simulink model "DataDriven_Sim"  (R2019a)
settings: Solver=ode4  StartTime=0.0  StopTime=40  FixedStep=0.005  MaxStep=0.2  RelTol=1e-3
values from neighbouring files (symbols this model uses):
  n = size(A,1)    [getMPC.m]    (also in poolData.m = size(yin,1); poolDataLIST.m = size(yin,1); poolData_EDMD.m = size(yin,1); solveMPCprob.m)
  nObsv = size(A,1)    [linearizeData.m]
  polyorder = p.polyorder    [sparseGalerkinControl_Discrete.m]
  polysine = p.polysine    [sparseGalerkinControl_Discrete.m]
  usesine = p.usesine    [sparseGalerkinControl_Discrete.m]
undefined symbols (not defined in the file or in its folder): F, Fi, lqi_, lqr_, param, ref_stab, ref_track, sigbuilder_block, stab, track
libraries: simulink x1
settings Model: Creator=yashasvi_sai  LastModifiedBy=ICS
settings SolverCC: ZeroCrossAlgorithm=Adaptive
settings DebuggingCC: IgnoredZcDiagnostic=none

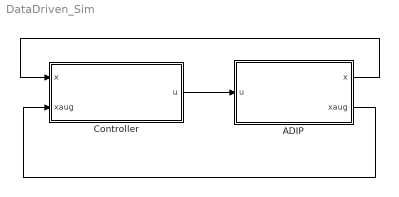
== system DataDriven_Sim ==
  ADIP : Subsystem
  Controller : Subsystem
  wires:
  ADIP/2(xaug) -> Controller/2(xaug)
  ADIP/1(x) -> Controller/1(x)
  Controller/1(u) -> ADIP/1(u)

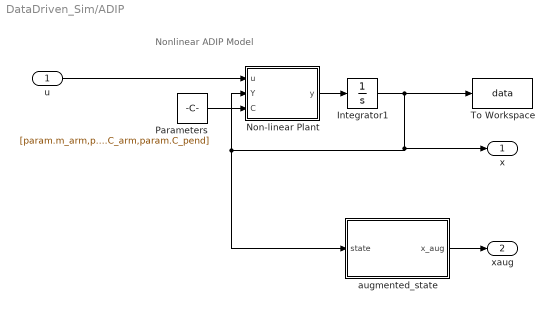
== system DataDriven_Sim/ADIP ==
  note: Nonlinear ADIP Model
  u : Inport
  Integrator1 : Integrator  InitialCondition=param.theta0
  "Non-linear Plant " : MATLAB Function  TreatAsAtomicUnit=on
  Parameters : Constant  Value=[param.m_arm,param.m_pend,param.m_hinge,param.l_pivot,param.l_pend,param.g,param.Jarm,param.Jpend,param.Jl,param.Jhinge, param.C_arm,param.C_pend]
  To Workspace : ToWorkspace  VariableName=data  SampleTime=-1
  augmented_state : Subsystem
  x : Outport
  xaug : Outport  Port=2
  wires:
  "Non-linear Plant "/1(y) -> Integrator1/1
  Integrator1/1 -> augmented_state/1(state), "Non-linear Plant "/2(Y), x/1, To Workspace/1
  u/1 -> "Non-linear Plant "/1(u)
  Parameters/1 -> "Non-linear Plant "/3(C)
  augmented_state/1(x_aug) -> xaug/1

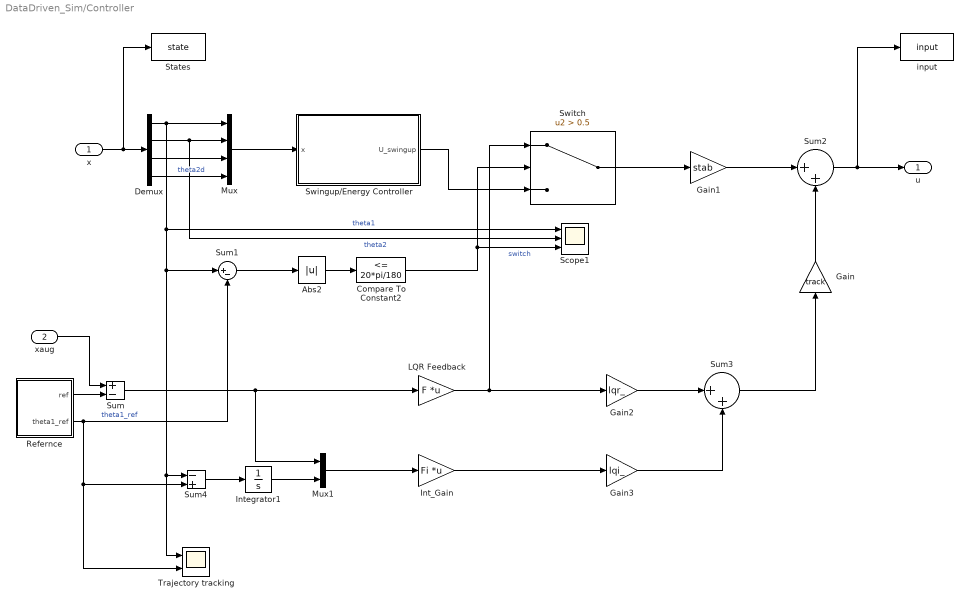
== system DataDriven_Sim/Controller ==
  x : Inport
  xaug : Inport  Port=2
  Abs2 : Abs
  Compare To Constant2 : simulink/Logic and Bit Operations/Compare To Constant  relop=<=  const=20*pi/180  OutDataTypeStr=boolean
  Demux : Demux
  Gain : Gain  Gain=track
  Gain1 : Gain  Gain=stab
  Gain2 : Gain  Gain=lqr_
  Gain3 : Gain  Gain=lqi_
  Int_Gain : Gain  Gain=Fi  Multiplication=Matrix(K*u)
  Integrator1 : Integrator
  LQR Feedback : Gain  Gain=F  Multiplication=Matrix(K*u)
  Mux : Mux
  Mux1 : Mux  Inputs=2
  Refernce : Subsystem
  Scope1 : Scope  NumInputPorts=3
  States : ToWorkspace  VariableName=state  SampleTime=-1
  Sum : Sum  Inputs=+-
  Sum1 : Sum  Inputs=|+-
  Sum2 : Sum  Inputs=|++
  Sum3 : Sum  Inputs=|++
  Sum4 : Sum  Inputs=-+
  Swingup/Energy Controller : Subsystem
  Switch : Switch  Criteria=u2 > Threshold  Threshold=0.5
  Trajectory tracking : Scope  NumInputPorts=2
  input : ToWorkspace  VariableName=input  SampleTime=-1
  u : Outport
  wires:
  x/1 -> States/1, Demux/1
  Swingup/Energy Controller/1(U_swingup) -> Switch/3
  Sum/1 -> LQR Feedback/1, Mux1/1
  Refernce/1(ref) -> Sum/2
  Abs2/1 -> Compare To Constant2/1
  Demux/3 -> Mux/3
  Demux/2 -> Scope1/2, Mux/2  "theta2"
  Demux/4 -> Mux/4  "theta2d"
  Mux/1 -> Swingup/Energy Controller/1(x)
  Sum1/1 -> Abs2/1
  Compare To Constant2/1 -> Scope1/3, Switch/2  "switch"
  xaug/1 -> Sum/1
  Demux/1 -> Scope1/1, Trajectory tracking/1, Sum4/1, Sum1/1, Mux/1  "theta1"
  Sum4/1 -> Integrator1/1
  Sum3/1 -> Gain/1
  Refernce/2(theta1_ref) -> Trajectory tracking/2, Sum4/2, Sum1/2  "theta1_ref"
  Integrator1/1 -> Mux1/2
  Gain/1 -> Sum2/2
  Gain1/1 -> Sum2/1
  Mux1/1 -> Int_Gain/1
  Switch/1 -> Gain1/1
  Sum2/1 -> input/1, u/1
  Gain2/1 -> Sum3/1
  LQR Feedback/1 -> Gain2/1, Switch/1
  Int_Gain/1 -> Gain3/1
  Gain3/1 -> Sum3/2

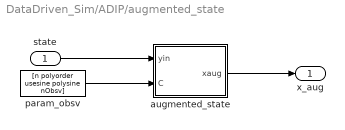
== system DataDriven_Sim/ADIP/augmented_state ==
  state : Inport
  augmented_state : MATLAB Function  TreatAsAtomicUnit=on
  param_obsv : Constant  Value=[n polyorder usesine polysine nObsv]
  x_aug : Outport
  wires:
  param_obsv/1 -> augmented_state/2(C)
  state/1 -> augmented_state/1(yin)
  augmented_state/1(xaug) -> x_aug/1

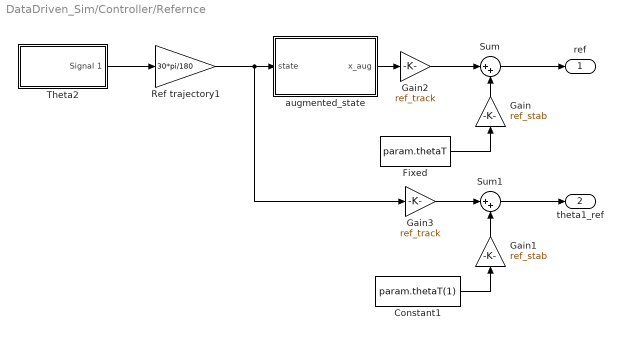
== system DataDriven_Sim/Controller/Refernce ==
  Constant1 : Constant  Value=param.thetaT(1)
  Fixed : Constant  Value=param.thetaT
  Gain : Gain  Gain=ref_stab
  Gain1 : Gain  Gain=ref_stab
  Gain2 : Gain  Gain=ref_track
  Gain3 : Gain  Gain=ref_track
  Ref trajectory1 : Gain  Gain=30*pi/180
  Sum : Sum  Inputs=|++
  Sum1 : Sum  Inputs=|++
  Theta2 : Subsystem  Tag=STV Subsys  LoadFcn=sigbuilder_block('load');  StartFcn=sigbuilder_block('start');  StopFcn=sigbuilder_block('stop');  ClipboardFcn=sigbuilder_block('clipboard');  mask(Sigbuilder block){tuvar=[0:10]}
      mask help: Simulink:masks:SigbuilderBlock_MD
      mask init:
      | if ~strcmp(get_param(bdroot(gcbh),'SimulationStatus'),'stopped') tuvar = sigbuilder_block('maskInit'); end
      settings: CopyFcn=sigbuilder_block('copy');  DeleteFcn=sigbuilder_block('delete');  ModelCloseFcn=sigbuilder_block('modelClose');  PreSaveFcn=sigbuilder_block('preSave');  PauseFcn=sigbuilder_block('pause');  ContinueFcn=sigbuilder_block('continue');  NameChangeFcn=sigbuilder_block('namechange');  OpenFcn=sigbuilder_block('open',[5.4 30 1141.2 522.6 ]);  CloseFcn=sigbuilder_block('close');
      mask Display: plot(0, 0, 100, 100,[2, 2, 32, 32, 2], [68, 8, 8, 68, 68],[32, 2], [38, 38], [32, 19, 2],[53, 60, 44], [32, 17, 17, 2],[16, 16, 31, 31]);txt = getActiveGroup(gcbh);text(2, 100, txt,'verticalAlignment', 'top');
  augmented_state : Subsystem
  ref : Outport
  theta1_ref : Outport  Port=2
  wires:
  Gain3/1 -> Sum1/1
  Gain2/1 -> Sum/1
  Gain/1 -> Sum/2
  Gain1/1 -> Sum1/2
  Fixed/1 -> Gain/1
  Ref trajectory1/1 -> augmented_state/1(state), Gain3/1
  Constant1/1 -> Gain1/1
  augmented_state/1(x_aug) -> Gain2/1
  Sum/1 -> ref/1
  Theta2/1(Signal 1) -> Ref trajectory1/1
  Sum1/1 -> theta1_ref/1

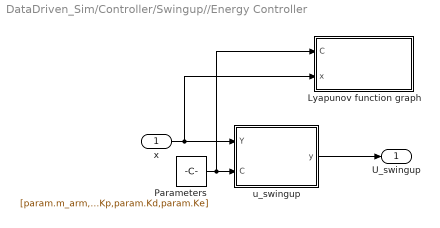
== system DataDriven_Sim/Controller/Swingup//Energy Controller ==
  x : Inport
  Lyapunov function graph : Subsystem
  Parameters : Constant  Value=[param.m_arm,param.m_pend,param.m_hinge,param.l_pivot,param.l_pend,param.g,param.Jarm,param.Jpend,param.Jl,param.Jhinge, param.C_arm,param.C_pend,param.Kp,param.Kd,param.Ke]
  "u_swingup " : MATLAB Function  TreatAsAtomicUnit=on
  U_swingup : Outport
  wires:
  x/1 -> Lyapunov function graph/2(x), "u_swingup "/1(Y)
  Parameters/1 -> Lyapunov function graph/1(C), "u_swingup "/2(C)
  "u_swingup "/1(y) -> U_swingup/1

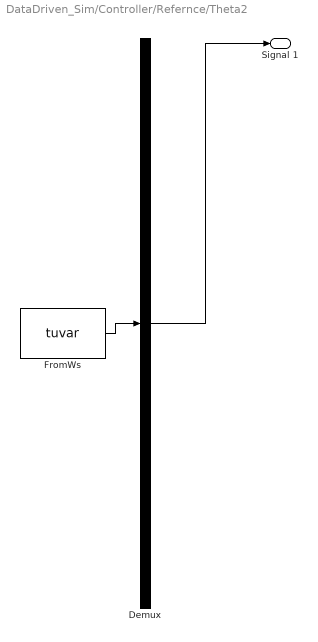
== system DataDriven_Sim/Controller/Refernce/Theta2 ==
  Demux : Demux  Tag=STV Demux  Outputs=1
  FromWs : FromWorkspace  Tag=STV FromWs  VariableName=tuvar  SampleTime=0
      SigBuilderData=|
      | common.afterFinalStr = 'Extrapolate'
      | common.sampleTime = 0
      | dataSet.timeRange = [0 50]
      | dataSet.name = 'Group 1'
      | sbobj.Groups.Name = 'Group 1'
      | sbobj.Groups.Signals.Name = 'Signal 1'
      | sbobj.Groups.Signals.XData = [0 8 11 15 20 25 28 40 50]
      | sbobj.Groups.Signals.YData = [0 0 1 1 -1 -1 0 0 0]
      | sbobj.Groups.TimeRange = [0 50]
  Signal 1 : Outport  Tag=STV Outport
  wires:
  Demux/1 -> Signal 1/1
  FromWs/1 -> Demux/1

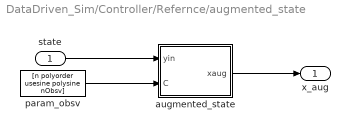
== system DataDriven_Sim/Controller/Refernce/augmented_state ==
  state : Inport
  augmented_state : MATLAB Function  TreatAsAtomicUnit=on
  param_obsv : Constant  Value=[n polyorder usesine polysine nObsv]
  x_aug : Outport
  wires:
  param_obsv/1 -> augmented_state/2(C)
  state/1 -> augmented_state/1(yin)
  augmented_state/1(xaug) -> x_aug/1

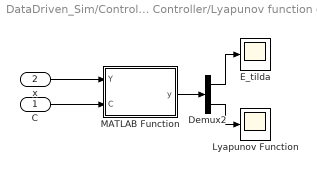
== system DataDriven_Sim/Controller/Swingup//Energy Controller/Lyapunov function graph ==
  C : Inport
  x : Inport  Port=2
  Demux2 : Demux  Outputs=2
  E_tilda : Scope
  Lyapunov Function : Scope
  MATLAB Function : MATLAB Function  TreatAsAtomicUnit=on
  wires:
  Demux2/1 -> E_tilda/1
  MATLAB Function/1(y) -> Demux2/1
  C/1 -> MATLAB Function/2(C)
  Demux2/2 -> Lyapunov Function/1
  x/1 -> MATLAB Function/1(Y)

== matlab function DataDriven_Sim/ADIP/Non-linear Plant  ==
  data: u input; Y input; y output; C input
function y = fcn(u,Y,C)
m1=C(1); % Mass of arm
m2=C(2); % Mass of pendulum
mh = C(3); % Mass of Hinge
l1  = C(4); % Length of arm
l2 = C(5); % Length of pendulum
g_ = C(6);
J_arm = C(7);
J_pend = C(8);
J_motor = C(9);
J_sensor = C(10);
fv1 = C(11);
fv2 = C(12);

y1 = Y(1);  % actual theta1          
y2 = Y(2);  % actual theta2
y3 = Y(3);  % actual theta1d
y4 = Y(4);  % actual theta2d

dy1 = y3;
dy2 = y4;
dy3 =-(2*(8*J_pend*fv1*y3 - 2*l2^2*m2*u - 8*J_pend*u + 2*fv1*l2^2*m2*y3 + l1^2*l2^2*m2^2*y3^2*sin(2*y1 - 2*y2) + l1*l2^3*m2^2*y4^2*sin(y1 - y2) + g_*l1*l2^2*m2^2*sin(y1) + 4*J_pend*g_*l1*m1*sin(y1) + 8*J_pend*g_*l1*m2*sin(y1) + 8*J_pend*g_*l1*mh*sin(y1) + g_*l1*l2^2*m2^2*sin(y1 - 2*y2) - 4*fv2*l1*l2*m2*y4*cos(y1 - y2) + g_*l1*l2^2*m1*m2*sin(y1) + 2*g_*l1*l2^2*m2*mh*sin(y1) + 4*J_pend*l1*l2*m2*y4^2*sin(y1 - y2)))/(16*J_arm*J_pend + 16*J_motor*J_pend + 16*J_pend*J_sensor + 4*l1^2*l2^2*m2^2 + 4*J_arm*l2^2*m2 + 4*J_motor*l2^2*m2 + 4*J_pend*l1^2*m1 + 16*J_pend*l1^2*m2 + 4*J_sensor*l2^2*m2 - 4*l1^2*l2^2*m2^2*cos(y1 - y2)^2 + l1^2*l2^2*m1*m2);
dy4 =(2*(l1^2*l2^2*m2^2*y4^2*sin(2*y1 - 2*y2) - 8*J_motor*fv2*y4 - 8*J_sensor*fv2*y4 - 2*fv2*l1^2*m1*y4 - 8*fv2*l1^2*m2*y4 - 8*J_arm*fv2*y4 - 4*l1*l2*m2*u*cos(y1 - y2) + 2*g_*l1^2*l2*m2^2*sin(2*y1 - y2) + 4*l1^3*l2*m2^2*y3^2*sin(y1 - y2) - 2*g_*l1^2*l2*m2^2*sin(y2) - 4*J_arm*g_*l2*m2*sin(y2) - 4*J_motor*g_*l2*m2*sin(y2) - 4*J_sensor*g_*l2*m2*sin(y2) + g_*l1^2*l2*m1*m2*sin(2*y1 - y2) + 2*g_*l1^2*l2*m2*mh*sin(2*y1 - y2) + l1^3*l2*m1*m2*y3^2*sin(y1 - y2) + 4*fv1*l1*l2*m2*y3*cos(y1 - y2) + 2*g_*l1^2*l2*m2*mh*sin(y2) + 4*J_arm*l1*l2*m2*y3^2*sin(y1 - y2) + 4*J_motor*l1*l2*m2*y3^2*sin(y1 - y2) + 4*J_sensor*l1*l2*m2*y3^2*sin(y1 - y2)))/(16*J_arm*J_pend + 16*J_motor*J_pend + 16*J_pend*J_sensor + 2*l1^2*l2^2*m2^2 + 4*J_arm*l2^2*m2 + 4*J_motor*l2^2*m2 + 4*J_pend*l1^2*m1 + 16*J_pend*l1^2*m2 + 4*J_sensor*l2^2*m2 - 2*l1^2*l2^2*m2^2*cos(2*y1 - 2*y2) + l1^2*l2^2*m1*m2);
y = [dy1 dy2 dy3 dy4]';

== matlab function DataDriven_Sim/ADIP/augmented_state/augmented_state ==
  data: yin input; xaug output; C input
function xaug = fcn(yin,C)

% % Manually entering the observables.
% y = [yin ;yin(1).^2 ;yin(1)*yin(2); yin(1)*yin(3); yin(1)*yin(4);yin(2).^2;...
%     yin(2)*yin(3); yin(2)*yin(4); yin(3).^2; yin(3)*yin(4); yin(4).^2]; 

yin = yin'; nVars = C(1); polyorder = C(2); usesine = C(3); polysine = C(4);
% nObsv = C(5);

y = zeros(1,34);
ind = 1;

% poly order 1
for i=1:nVars
    y(:,ind) = yin(:,i);
    ind = ind+1;
end

if(polyorder>=2)
    % poly order 2
    for i=1:nVars
        for j=i:nVars
            y(:,ind) = yin(:,i).*yin(:,j);
            ind = ind+1;
        end
    end
end

xaug = y';


% n = size(yin,1);
% yout = zeros(1,4);
% ind = 1;
% % poly order 0
% % yout(:,ind) = ones(n,1);
% % ind = ind+1;
% 

% 

% 
% if(polyorder>=3)
%     % poly order 3
%     for i=1:nVars
%         for j=i:nVars
%             for k=j:nVars
%                 yout(:,ind) = yin(:,i).*yin(:,j).*yin(:,k);
%                 ind = ind+1;
%             end
%         end
%     end
% end
% 
% if(polyorder>=4)
%     % poly order 4
%     for i=1:nVars
%         for j=i:nVars
%             for k=j:nVars
%                 for l=k:nVars
%                     yout(:,ind) = yin(:,i).*yin(:,j).*yin(:,k).*yin(:,l);
%                     ind = ind+1;
%                 end
%             end
%         end
%     end
% end
% 
% if(polyorder>=5)
%     % poly order 5
%     for i=1:nVars
%         for j=i:nVars
%             for k=j:nVars
%                 for l=k:nVars
%                     for m=l:nVars
%                         yout(:,ind) = yin(:,i).*yin(:,j).*yin(:,k).*yin(:,l).*yin(:,m);
%                         ind = ind+1;
%                     end
%                 end
%             end
%         end
%     end
% end
% 
% % if(usesine)
% %     for k=1:10
% %         yout = [yout sin(k*yin) cos(k*yin)];
% %     end
% % end
% % 
% % if(polysine)
% %     for i=1:nVars
% %         for k= 1:10
% %             yout = [yout yin(:,i).*sin(k*yin) yin(:,i).*cos(k*yin)];
% %         end
% %     end
% % end
% 
% if(usesine)
%     for k=1:2
%         yout = [yout sin(k*yin(:,1:2)) cos(k*yin(:,1:2))];
%     end
% end
% 
% if(polysine)
%     for i=1:nVars
%         for k= 1:2
%             yout = [yout yin(:,i).*sin(k*yin(:,1:2)) yin(:,i).*cos(k*yin(:,1:2))];
%         end
%     end
% end
% 
% if(polysine)
%     for i=1:nVars
%         for j= 1:nVars
%             for k= 1:2
%                 yout = [yout yin(:,i).*yin(:,j).*sin(k*yin(:,1:2)) yin(:,i).*yin(:,j).*cos(k*yin(:,1:2))];
%             end
%         end
%     end
% end
% 
% y = yout';

== matlab function DataDriven_Sim/Controller/Refernce/augmented_state/augmented_state ==
  data: yin input; xaug output; C input
function xaug = fcn(yin,C)

% % Manually entering the observables.
% y = [yin ;yin(1).^2 ;yin(1)*yin(2); yin(1)*yin(3); yin(1)*yin(4);yin(2).^2;...
%     yin(2)*yin(3); yin(2)*yin(4); yin(3).^2; yin(3)*yin(4); yin(4).^2]; 

yin = [yin ;0 ;0 ;0]'; 
nVars = C(1); polyorder = C(2); usesine = C(3); polysine = C(4);
% nObsv = C(5);

y = zeros(1,34);
ind = 1;

% poly order 1
for i=1:nVars
    y(:,ind) = yin(:,i);
    ind = ind+1;
end

if(polyorder>=2)
    % poly order 2
    for i=1:nVars
        for j=i:nVars
            y(:,ind) = yin(:,i).*yin(:,j);
            ind = ind+1;
        end
    end
end

xaug = y';


% n = size(yin,1);
% yout = zeros(1,4);
% ind = 1;
% % poly order 0
% % yout(:,ind) = ones(n,1);
% % ind = ind+1;
% 

% 

% 
% if(polyorder>=3)
%     % poly order 3
%     for i=1:nVars
%         for j=i:nVars
%             for k=j:nVars
%                 yout(:,ind) = yin(:,i).*yin(:,j).*yin(:,k);
%                 ind = ind+1;
%             end
%         end
%     end
% end
% 
% if(polyorder>=4)
%     % poly order 4
%     for i=1:nVars
%         for j=i:nVars
%             for k=j:nVars
%                 for l=k:nVars
%                     yout(:,ind) = yin(:,i).*yin(:,j).*yin(:,k).*yin(:,l);
%                     ind = ind+1;
%                 end
%             end
%         end
%     end
% end
% 
% if(polyorder>=5)
%     % poly order 5
%     for i=1:nVars
%         for j=i:nVars
%             for k=j:nVars
%                 for l=k:nVars
%                     for m=l:nVars
%                         yout(:,ind) = yin(:,i).*yin(:,j).*yin(:,k).*yin(:,l).*yin(:,m);
%                         ind = ind+1;
%                     end
%                 end
%             end
%         end
%     end
% end
% 
% % if(usesine)
% %     for k=1:10
% %         yout = [yout sin(k*yin) cos(k*yin)];
% %     end
% % end
% % 
% % if(polysine)
% %     for i=1:nVars
% %         for k= 1:10
% %             yout = [yout yin(:,i).*sin(k*yin) yin(:,i).*cos(k*yin)];
% %         end
% %     end
% % end
% 
% if(usesine)
%     for k=1:2
%         yout = [yout sin(k*yin(:,1:2)) cos(k*yin(:,1:2))];
%     end
% end
% 
% if(polysine)
%     for i=1:nVars
%         for k= 1:2
%             yout = [yout yin(:,i).*sin(k*yin(:,1:2)) yin(:,i).*cos(k*yin(:,1:2))];
%         end
%     end
% end
% 
% if(polysine)
%     for i=1:nVars
%         for j= 1:nVars
%             for k= 1:2
%                 yout = [yout yin(:,i).*yin(:,j).*sin(k*yin(:,1:2)) yin(:,i).*yin(:,j).*cos(k*yin(:,1:2))];
%             end
%         end
%     end
% end
% 
% y = yout';

== matlab function DataDriven_Sim/Controller/Swingup//Energy Controller/Lyapunov function graph/MATLAB Function ==
  data: Y input; y output; C input
function y = fcn(Y,C)

m1=C(1); % Mass of arm
m2=C(2); % Mass of pendulum
mh = C(3); % Mass of Hinge
l1  = C(4); % Length of arm
l2 = C(5); % Length of pendulum
g_ = C(6);
J_arm = C(7);
J_pend = C(8);
J_motor = C(9);
J_sensor = C(10);
fv1 = C(11);
fv2 = C(12);

y1 = Y(1);  % actual theta1          
y2 = Y(2);  % actual theta2
y3 = Y(3);  % actual theta1d
y4 = Y(4);  % actual theta2d

Kp = C(13);
Kd = C(14);
Ke = C(15);

y1_tilda = Y(1);

E_tilda = (J_arm*y3^2)/2 + (J_motor*y3^2)/2 + (J_pend*y4^2)/2 + (J_sensor*y3^2)/2 + g_*m1*(l1/2 - (l1*cos(y1))/2) + g_*m2*(l1 + l2/2 - l1*cos(y1) - (l2*cos(y2))/2) + g_*mh*(l1 - l1*cos(y1));
V_L = 0.5*(Ke*E_tilda^2 + Kd*y3^2 + Kp*(y1_tilda)^2);

y = [E_tilda V_L];

== matlab function DataDriven_Sim/Controller/Swingup//Energy Controller/u_swingup  ==
  data: Y input; y output; C input
function y = fcn(Y, C)
m1=C(1); % Mass of arm
m2=C(2); % Mass of pendulum
mh = C(3); % Mass of Hinge
l1  = C(4); % Length of arm
l2 = C(5); % Length of pendulum
g_ = C(6);
J_arm = C(7);
J_pend = C(8);
J_motor = C(9);
J_sensor = C(10);
fv1 = C(11);
fv2 = C(12);

y1 = Y(1);  % actual theta1          
y2 = Y(2);  % actual theta2
y3 = Y(3);  % actual theta1d
y4 = Y(4);  % actual theta2d

Kp = C(13);
Kd = C(14);
Ke = C(15);

y1_tilda = Y(1);

u_swing = (Kd*(J_pend*fv1*y3 + (fv1*l2^2*m2*y3)/4 + (l1^2*l2^2*m2^2*y3^2*sin(2*y1 - 2*y2))/8 + (l1*l2^3*m2^2*y4^2*sin(y1 - y2))/8 + (g_*l1*l2^2*m2^2*sin(y1))/8 + (J_pend*g_*l1*m1*sin(y1))/2 + J_pend*g_*l1*m2*sin(y1) + J_pend*g_*l1*mh*sin(y1) + (g_*l1*l2^2*m2^2*sin(y1 - 2*y2))/8 - (fv2*l1*l2*m2*y4*cos(y1 - y2))/2 + (g_*l1*l2^2*m1*m2*sin(y1))/8 + (g_*l1*l2^2*m2*mh*sin(y1))/4 + (J_pend*l1*l2*m2*y4^2*sin(y1 - y2))/2) - (y3 + Kp*y1_tilda)*(J_arm*J_pend + J_motor*J_pend + J_pend*J_sensor + (l1^2*l2^2*m2^2)/4 + (J_arm*l2^2*m2)/4 + (J_motor*l2^2*m2)/4 + (J_pend*l1^2*m1)/4 + J_pend*l1^2*m2 + (J_sensor*l2^2*m2)/4 - (l1^2*l2^2*m2^2*cos(y1 - y2)^2)/4 + (l1^2*l2^2*m1*m2)/16))/(Kd*((m2*l2^2)/4 + J_pend) + Ke*((J_arm*y3^2)/2 + (J_motor*y3^2)/2 + (J_pend*y4^2)/2 + (J_sensor*y3^2)/2 + g_*m1*(l1/2 - (l1*cos(y1))/2) + g_*m2*(l1 + l2/2 - l1*cos(y1) - (l2*cos(y2))/2) + g_*mh*(l1 - l1*cos(y1)))*(J_arm*J_pend + J_motor*J_pend + J_pend*J_sensor + (l1^2*l2^2*m2^2)/4 + (J_arm*l2^2*m2)/4 + (J_motor*l2^2*m2)/4 + (J_pend*l1^2*m1)/4 + J_pend*l1^2*m2 + (J_sensor*l2^2*m2)/4 - (l1^2*l2^2*m2^2*cos(y1 - y2)^2)/4 + (l1^2*l2^2*m1*m2)/16));
y = u_swing;
